simulink model "version1"  (R2021a)
settings: Solver=ode4  StartTime=0.0  StopTime=10.0  FixedStep=1e-6  RelTol=1e-3
settings Model: Creator=Aashish Kalra  LastModifiedBy=Aashish Kalra

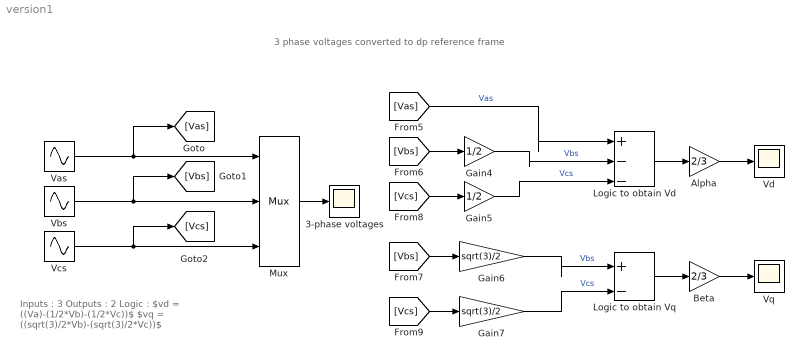
== system version1 ==
  note: Inputs : 3
      | Outputs : 2
      |
      | Logic :
      | $vd = ((Va)-(1/2*Vb)-(1/2*Vc))$
      | $vq = ((sqrt(3)/2*Vb)-(sqrt(3)/2*Vc))$
  note: 3 phase voltages converted to dp reference frame
  3-phase voltages : Scope
  Alpha : Gain  Gain=2/3
  Beta : Gain  Gain=2/3
  Gain4 : Gain  Gain=1/2
  Gain5 : Gain  Gain=1/2
  Gain6 : Gain  Gain=sqrt(3)/2
  Gain7 : Gain  Gain=sqrt(3)/2
  Logic to obtain Vd : Sum  Inputs=|+--
  Logic to obtain Vq : Sum  Inputs=|+-
  Mux : Mux  Inputs=3
  Vas : Sin  Amplitude=220*sqrt(2)  Frequency=2*pi*60  Phase=(pi/2)  SampleTime=0
  Vbs : Sin  Amplitude=220*sqrt(2)  Frequency=2*pi*60  Phase=((-2*pi)/3)+(pi/2)  SampleTime=0
  Vcs : Sin  Amplitude=220*sqrt(2)  Frequency=2*pi*60  Phase=((2*pi)/3)+(pi/2)  SampleTime=0
  Vd : Scope
  Vq : Scope
  wires:
  Gain7/1 -> Logic to obtain Vq/2  "Vcs"
  [Vcs] -> Gain5/1
  Beta/1 -> Vq/1
  Gain5/1 -> Logic to obtain Vd/3  "Vcs"
  Logic to obtain Vd/1 -> Alpha/1
  [Vas] -> Logic to obtain Vd/1  "Vas"
  Gain6/1 -> Logic to obtain Vq/1  "Vbs"
  [Vcs] -> Gain7/1
  Logic to obtain Vq/1 -> Beta/1
  Alpha/1 -> Vd/1
  Gain4/1 -> Logic to obtain Vd/2  "Vbs"
  [Vbs] -> Gain6/1
  [Vbs] -> Gain4/1
  Vbs/1 -> [Vbs], Mux/2
  Vcs/1 -> [Vcs], Mux/3
  Vas/1 -> [Vas], Mux/1
  Mux/1 -> 3-phase voltages/1
